simulink library "lib_ThermalManager"  (R2017a)
settings: Solver=VariableStepAuto  StartTime=0.0  StopTime=10.0  RelTol=1e-3
undefined symbols (not defined in the file): c
libraries: simulink x12
settings Model: Creator=Di Russo  LastModifiedBy=Di Russo

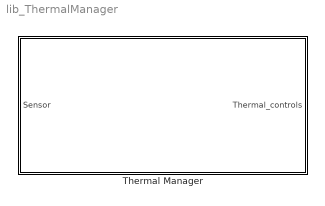
== system lib_ThermalManager ==
  Thermal Manager : Subsystem

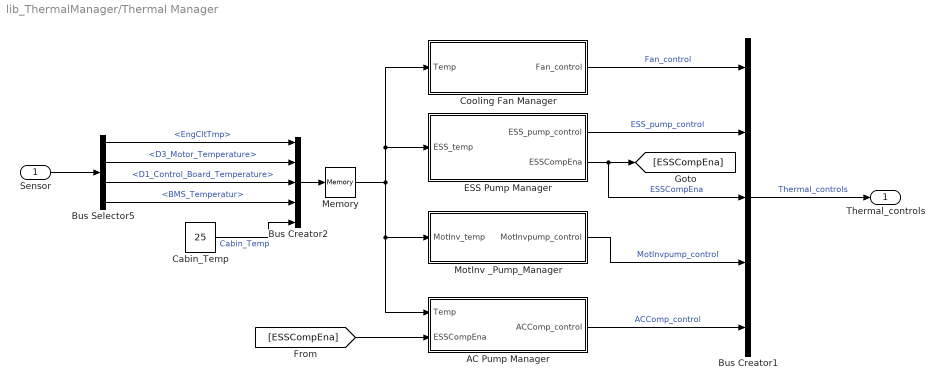
== system lib_ThermalManager/Thermal Manager ==
  Sensor : Inport
  AC Pump Manager : Subsystem
  Bus Creator1 : BusCreator  Inputs=5
  Bus Creator2 : BusCreator  Inputs=5
  Bus Selector5 : BusSelector  OutputSignals=from_CAN.fromEBCAN.from_ECM.EngCltTmp,from_CAN.fromHV_CAN.from_MCU.D3_Motor_Temperature,from_CAN.fromHV_CAN.from_MCU.D1_Control_Board_Temperature,from_CAN.fromHV_CAN.from_BMSHybrid.BMS_Temperatur
  Cabin_Temp : Constant  Value=25
  Cooling Fan Manager : Subsystem
  ESS Pump Manager : Subsystem
  Memory : Memory  X0=25
  MotInv _Pump_Manager : Subsystem
  Thermal_controls : Outport
  wires:
  Bus Creator1/1 -> Thermal_controls/1  "Thermal_controls"
  ESS Pump Manager/1(ESS_pump_control) -> Bus Creator1/2  "ESS_pump_control"
  Cooling Fan Manager/1(Fan_control) -> Bus Creator1/1  "Fan_control"
  Bus Creator2/1 -> Memory/1
  AC Pump Manager/1(ACComp_control) -> Bus Creator1/5  "ACComp_control"
  MotInv _Pump_Manager/1(MotInvpump_control) -> Bus Creator1/4  "MotInvpump_control"
  Bus Selector5/1 -> Bus Creator2/1  "<EngCltTmp>"
  Bus Selector5/2 -> Bus Creator2/2  "<D3_Motor_Temperature>"
  Bus Selector5/3 -> Bus Creator2/3  "<D1_Control_Board_Temperature>"
  Bus Selector5/4 -> Bus Creator2/4  "<BMS_Temperatur>"
  Sensor/1 -> Bus Selector5/1
  Cabin_Temp/1 -> Bus Creator2/5  "Cabin_Temp"
  ESS Pump Manager/2(ESSCompEna) -> Bus Creator1/3, [ESSCompEna]  "ESSCompEna"
  [ESSCompEna] -> AC Pump Manager/2(ESSCompEna)
  Memory/1 -> AC Pump Manager/1(Temp), MotInv _Pump_Manager/1(MotInv_temp), Cooling Fan Manager/1(Temp), ESS Pump Manager/1(ESS_temp)

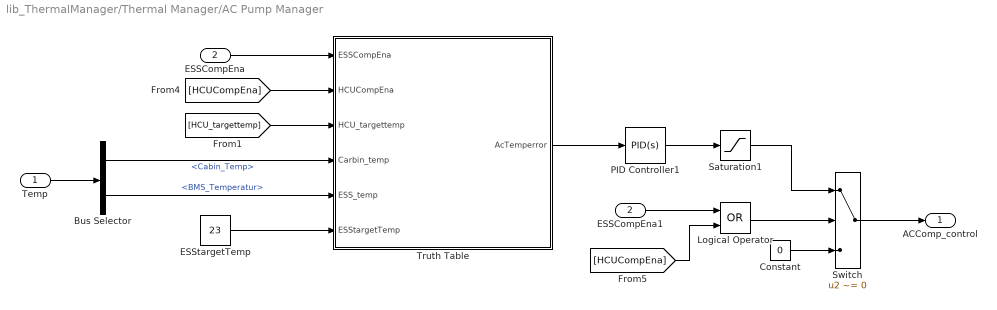
== system lib_ThermalManager/Thermal Manager/AC Pump Manager ==
  Temp : Inport
  ESSCompEna : Inport  Port=2
  Bus Selector : BusSelector  OutputSignals=Cabin_Temp,BMS_Temperatur
  Constant : Constant  Value=0
  ESSCompEna1 : InportShadow  Port=2
  ESStargetTemp : Constant  Value=23
  Logical Operator : Logic  Operator=OR  AllPortsSameDT=off  OutDataTypeStr=boolean
  PID Controller1 : simulink/Continuous/PID Controller  Controller=PID  TimeDomain=Continuous-time  SampleTime=-1  IntegratorMethod=Forward Euler  FilterMethod=Forward Euler  Form=Parallel  UseFilter=on  ControllerParametersSource=internal  P=1  I=0.01  D=0  N=100  InitialConditionSource=internal  InitialConditionForIntegrator=0  InitialConditionForFilter=0  ExternalReset=none  LimitOutput=off  UpperSaturationLimit=inf  LowerSaturationLimit=-inf  LinearizeAsGain=on  AntiWindupMode=none  Kb=1  TrackingMode=off  Kt=1  PParamMin=[]  PParamMax=[]  IParamMin=[]  IParamMax=[]  DParamMin=[]  DParamMax=[]  NParamMin=[]  NParamMax=[]  KbParamMin=[]  KbParamMax=[]  KtParamMin=[]  KtParamMax=[]  POutMin=[]  POutMax=[]  IOutMin=[]  IOutMax=[]  DOutMin=[]  DOutMax=[]  NOutMin=[]  NOutMax=[]  KbOutMin=[]  KbOutMax=[]  KtOutMin=[]  KtOutMax=[]  IntegratorOutMin=[]  IntegratorOutMax=[]  FilterOutMin=[]  FilterOutMax=[]  SumOutMin=[]  SumOutMax=[]  SumI1OutMin=[]  SumI1OutMax=[]  SumI2OutMin=[]  SumI2OutMax=[]  SumI3OutMin=[]  SumI3OutMax=[]  SumDOutMin=[]  SumDOutMax=[]  SaturationOutMin=[]  SaturationOutMax=[]  IntegratorContinuousStateAttributes=''  IntegratorStateMustResolveToSignalObject=off  IntegratorRTWStateStorageClass=Auto  FilterContinuousStateAttributes=''  FilterStateMustResolveToSignalObject=off  FilterRTWStateStorageClass=Auto  DifferentiatorICPrevScaledInput=0  DifferentiatorOutMin=[]  DifferentiatorOutMax=[]  InitialConditionSetting=State (most efficient)
  Saturation1 : Saturate  UpperLimit=1  LowerLimit=0.094
  Switch : Switch  Criteria=u2 ~= 0
  Truth Table : Truth Table  TreatAsAtomicUnit=on
  ACComp_control : Outport
  wires:
  Temp/1 -> Bus Selector/1
  PID Controller1/1 -> Saturation1/1
  Bus Selector/1 -> Truth Table/4(Carbin_temp)  "<Cabin_Temp>"
  Bus Selector/2 -> Truth Table/5(ESS_temp)  "<BMS_Temperatur>"
  ESStargetTemp/1 -> Truth Table/6(ESStargetTemp)
  Truth Table/1(AcTemperror) -> PID Controller1/1
  ESSCompEna/1 -> Truth Table/1(ESSCompEna)
  Logical Operator/1 -> Switch/2
  Constant/1 -> Switch/3
  Saturation1/1 -> Switch/1
  Switch/1 -> ACComp_control/1
  [HCU_targettemp] -> Truth Table/3(HCU_targettemp)
  [HCUCompEna] -> Truth Table/2(HCUCompEna)
  [HCUCompEna] -> Logical Operator/2
  ESSCompEna1/1 -> Logical Operator/1

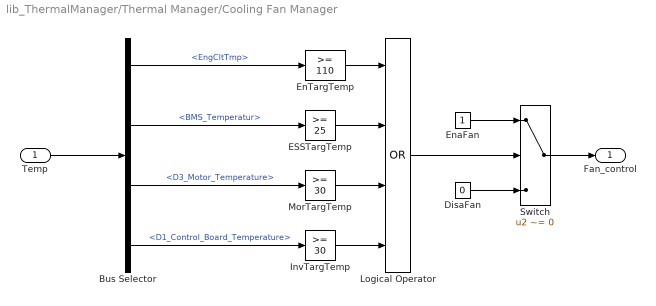
== system lib_ThermalManager/Thermal Manager/Cooling Fan Manager ==
  Temp : Inport
  Bus Selector : BusSelector  OutputSignals=EngCltTmp,BMS_Temperatur,D3_Motor_Temperature,D1_Control_Board_Temperature
  DisaFan : Constant  Value=0
  ESSTargTemp : simulink/Logic and Bit Operations/Compare To Constant  relop=>=  const=25  OutDataTypeStr=boolean
  EnTargTemp : simulink/Logic and Bit Operations/Compare To Constant  relop=>=  const=110  OutDataTypeStr=boolean
  EnaFan : Constant
  InvTargTemp : simulink/Logic and Bit Operations/Compare To Constant  relop=>=  const=30  OutDataTypeStr=boolean
  Logical Operator : Logic  Operator=OR  Inputs=4  AllPortsSameDT=off  OutDataTypeStr=boolean
  MorTargTemp : simulink/Logic and Bit Operations/Compare To Constant  relop=>=  const=30  OutDataTypeStr=boolean
  Switch : Switch  Criteria=u2 ~= 0
  Fan_control : Outport
  wires:
  Temp/1 -> Bus Selector/1
  Switch/1 -> Fan_control/1
  DisaFan/1 -> Switch/3
  Logical Operator/1 -> Switch/2
  EnaFan/1 -> Switch/1
  Bus Selector/1 -> EnTargTemp/1  "<EngCltTmp>"
  Bus Selector/2 -> ESSTargTemp/1  "<BMS_Temperatur>"
  Bus Selector/3 -> MorTargTemp/1  "<D3_Motor_Temperature>"
  Bus Selector/4 -> InvTargTemp/1  "<D1_Control_Board_Temperature>"
  EnTargTemp/1 -> Logical Operator/1
  ESSTargTemp/1 -> Logical Operator/2
  MorTargTemp/1 -> Logical Operator/3
  InvTargTemp/1 -> Logical Operator/4

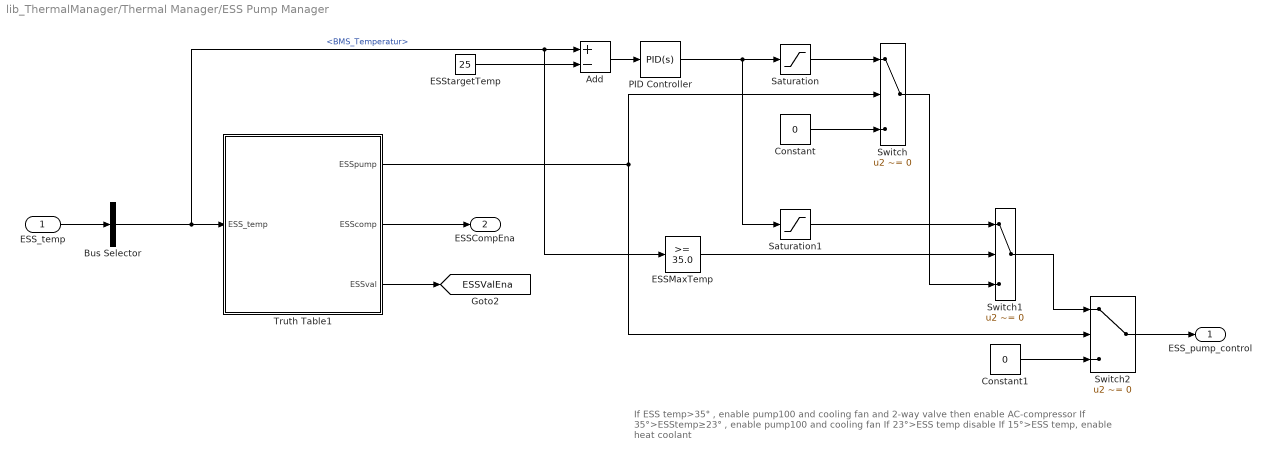
== system lib_ThermalManager/Thermal Manager/ESS Pump Manager ==
  note: If ESS temp>35°，enable pump100 and cooling fan and 2-way valve then enable AC-compressor
      |
      | If 35°>ESStemp≥23°，enable pump100 and cooling fan
      |
      | If 23°>ESS temp disable
      |
      | If 15°>ESS temp, enable heat coolant
  ESS_temp : Inport
  Add : Sum  Inputs=+-
  Bus Selector : BusSelector  OutputSignals=BMS_Temperatur
  Constant : Constant  Value=0
  Constant1 : Constant  Value=0
  ESSMaxTemp : simulink/Logic and Bit Operations/Compare To Constant  relop=>=  const=35.0  OutDataTypeStr=boolean
  ESStargetTemp : Constant  Value=25
  PID Controller : simulink/Continuous/PID Controller  Controller=PID  TimeDomain=Continuous-time  SampleTime=-1  IntegratorMethod=Forward Euler  FilterMethod=Forward Euler  Form=Parallel  UseFilter=on  ControllerParametersSource=internal  P=1  I=0.01  D=0  N=100  InitialConditionSource=internal  InitialConditionForIntegrator=0  InitialConditionForFilter=0  ExternalReset=none  LimitOutput=off  UpperSaturationLimit=inf  LowerSaturationLimit=-inf  LinearizeAsGain=on  AntiWindupMode=none  Kb=1  TrackingMode=off  Kt=1  PParamMin=[]  PParamMax=[]  IParamMin=[]  IParamMax=[]  DParamMin=[]  DParamMax=[]  NParamMin=[]  NParamMax=[]  KbParamMin=[]  KbParamMax=[]  KtParamMin=[]  KtParamMax=[]  POutMin=[]  POutMax=[]  IOutMin=[]  IOutMax=[]  DOutMin=[]  DOutMax=[]  NOutMin=[]  NOutMax=[]  KbOutMin=[]  KbOutMax=[]  KtOutMin=[]  KtOutMax=[]  IntegratorOutMin=[]  IntegratorOutMax=[]  FilterOutMin=[]  FilterOutMax=[]  SumOutMin=[]  SumOutMax=[]  SumI1OutMin=[]  SumI1OutMax=[]  SumI2OutMin=[]  SumI2OutMax=[]  SumI3OutMin=[]  SumI3OutMax=[]  SumDOutMin=[]  SumDOutMax=[]  SaturationOutMin=[]  SaturationOutMax=[]  IntegratorContinuousStateAttributes=''  IntegratorStateMustResolveToSignalObject=off  IntegratorRTWStateStorageClass=Auto  FilterContinuousStateAttributes=''  FilterStateMustResolveToSignalObject=off  FilterRTWStateStorageClass=Auto  DifferentiatorICPrevScaledInput=0  DifferentiatorOutMin=[]  DifferentiatorOutMax=[]  InitialConditionSetting=State (most efficient)
  Saturation : Saturate  UpperLimit=0.85  LowerLimit=0.13
  Saturation1 : Saturate  UpperLimit=0.97  LowerLimit=0.86
  Switch : Switch  Criteria=u2 ~= 0
  Switch1 : Switch  Criteria=u2 ~= 0  Threshold=1
  Switch2 : Switch  Criteria=u2 ~= 0  Threshold=c
  Truth Table1 : Truth Table  TreatAsAtomicUnit=on
  ESS_pump_control : Outport
  ESSCompEna : Outport  Port=2
  tag scope: ESSValEna=global
  wires:
  Truth Table1/1(ESSpump) -> Switch2/2, Switch/2
  ESS_temp/1 -> Bus Selector/1
  Bus Selector/1 -> ESSMaxTemp/1, Add/1, Truth Table1/1(ESS_temp)  "<BMS_Temperatur>"
  Constant/1 -> Switch/3
  PID Controller/1 -> Saturation1/1, Saturation/1
  Add/1 -> PID Controller/1
  Saturation/1 -> Switch/1
  ESSMaxTemp/1 -> Switch1/2
  ESStargetTemp/1 -> Add/2
  Truth Table1/2(ESScomp) -> ESSCompEna/1
  Truth Table1/3(ESSval) -> [ESSValEna]
  Constant1/1 -> Switch2/3
  Switch2/1 -> ESS_pump_control/1
  Switch1/1 -> Switch2/1
  Switch/1 -> Switch1/3
  Saturation1/1 -> Switch1/1

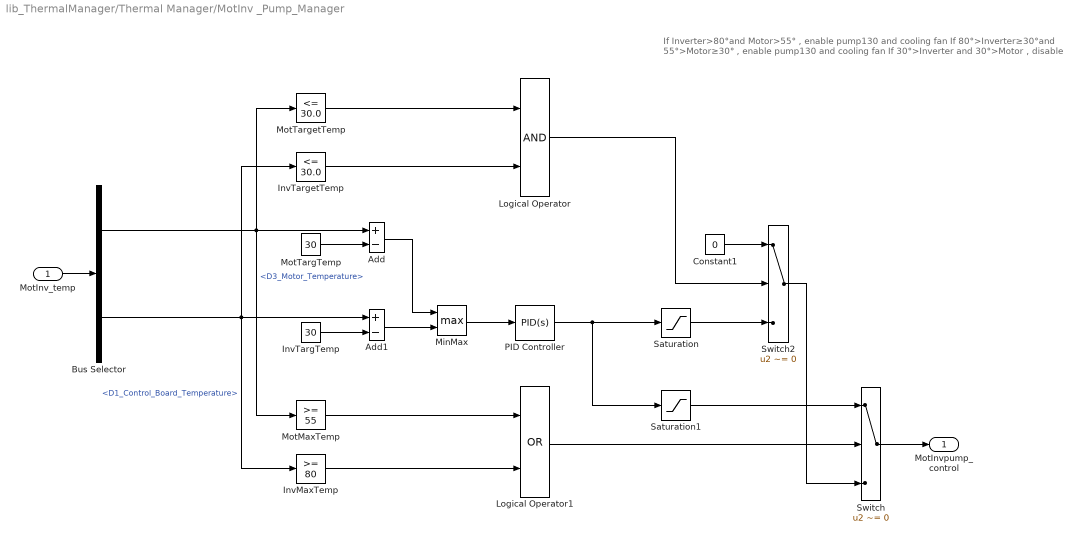
== system lib_ThermalManager/Thermal Manager/MotInv _Pump_Manager ==
  note: If Inverter>80°and Motor>55°，enable pump130 and cooling fan
      |
      | If 80°>Inverter≥30°and 55°>Motor≥30°，enable pump130 and cooling fan
      |
      | If 30°>Inverter and 30°>Motor，disable
  MotInv_temp : Inport
  Add : Sum  Inputs=+-
  Add1 : Sum  Inputs=+-
  Bus Selector : BusSelector  OutputSignals=D3_Motor_Temperature,D1_Control_Board_Temperature
  Constant1 : Constant  Value=0
  InvMaxTemp : simulink/Logic and Bit Operations/Compare To Constant  relop=>=  const=80  OutDataTypeStr=boolean
  InvTargTemp : Constant  Value=30
  InvTargetTemp : simulink/Logic and Bit Operations/Compare To Constant  relop=<=  const=30.0  OutDataTypeStr=boolean
  Logical Operator : Logic  AllPortsSameDT=off  OutDataTypeStr=boolean
  Logical Operator1 : Logic  Operator=OR  AllPortsSameDT=off  OutDataTypeStr=boolean
  MinMax : MinMax  Function=max  Inputs=2
  MotMaxTemp : simulink/Logic and Bit Operations/Compare To Constant  relop=>=  const=55  OutDataTypeStr=boolean
  MotTargTemp : Constant  Value=30
  MotTargetTemp : simulink/Logic and Bit Operations/Compare To Constant  relop=<=  const=30.0  OutDataTypeStr=boolean
  PID Controller : simulink/Continuous/PID Controller  Controller=PID  TimeDomain=Continuous-time  SampleTime=-1  IntegratorMethod=Forward Euler  FilterMethod=Forward Euler  Form=Parallel  UseFilter=on  ControllerParametersSource=internal  P=0.05  I=0.001  D=5  N=100  InitialConditionSource=internal  InitialConditionForIntegrator=0  InitialConditionForFilter=0  ExternalReset=none  LimitOutput=off  UpperSaturationLimit=inf  LowerSaturationLimit=-inf  LinearizeAsGain=on  AntiWindupMode=none  Kb=1  TrackingMode=off  Kt=1  PParamMin=[]  PParamMax=[]  IParamMin=[]  IParamMax=[]  DParamMin=[]  DParamMax=[]  NParamMin=[]  NParamMax=[]  KbParamMin=[]  KbParamMax=[]  KtParamMin=[]  KtParamMax=[]  POutMin=[]  POutMax=[]  IOutMin=[]  IOutMax=[]  DOutMin=[]  DOutMax=[]  NOutMin=[]  NOutMax=[]  KbOutMin=[]  KbOutMax=[]  KtOutMin=[]  KtOutMax=[]  IntegratorOutMin=[]  IntegratorOutMax=[]  FilterOutMin=[]  FilterOutMax=[]  SumOutMin=[]  SumOutMax=[]  SumI1OutMin=[]  SumI1OutMax=[]  SumI2OutMin=[]  SumI2OutMax=[]  SumI3OutMin=[]  SumI3OutMax=[]  SumDOutMin=[]  SumDOutMax=[]  SaturationOutMin=[]  SaturationOutMax=[]  IntegratorContinuousStateAttributes=''  IntegratorStateMustResolveToSignalObject=off  IntegratorRTWStateStorageClass=Auto  FilterContinuousStateAttributes=''  FilterStateMustResolveToSignalObject=off  FilterRTWStateStorageClass=Auto  DifferentiatorICPrevScaledInput=0  DifferentiatorOutMin=[]  DifferentiatorOutMax=[]  InitialConditionSetting=State (most efficient)
  Saturation : Saturate  UpperLimit=0.85  LowerLimit=0.13
  Saturation1 : Saturate  UpperLimit=0.97  LowerLimit=0.86
  Switch : Switch  Criteria=u2 ~= 0  Threshold=1
  Switch2 : Switch  Criteria=u2 ~= 0  Threshold=1
  MotInvpump_control : Outport
  wires:
  MotInv_temp/1 -> Bus Selector/1
  Bus Selector/1 -> MotTargetTemp/1, Add/1, MotMaxTemp/1  "<D3_Motor_Temperature>"
  Bus Selector/2 -> InvTargetTemp/1, InvMaxTemp/1, Add1/1  "<D1_Control_Board_Temperature>"
  MotTargetTemp/1 -> Logical Operator/1
  InvTargetTemp/1 -> Logical Operator/2
  Add/1 -> MinMax/1
  Add1/1 -> MinMax/2
  MinMax/1 -> PID Controller/1
  PID Controller/1 -> Saturation1/1, Saturation/1
  Logical Operator/1 -> Switch2/2
  MotMaxTemp/1 -> Logical Operator1/1
  InvMaxTemp/1 -> Logical Operator1/2
  Logical Operator1/1 -> Switch/2
  Switch/1 -> MotInvpump_control/1
  MotTargTemp/1 -> Add/2
  InvTargTemp/1 -> Add1/2
  Switch2/1 -> Switch/3
  Saturation1/1 -> Switch/1
  Saturation/1 -> Switch2/3
  Constant1/1 -> Switch2/1

== matlab function lib_ThermalManager/Thermal Manager/AC Pump Manager/Truth Table ==
  data: ESSCompEna input; AcTemperror output; HCUCompEna input double; HCU_targettemp input double; Carbin_temp input double; ESS_temp input double; ESStargetTemp input double
function AcTemperror = fcn(ESSCompEna, HCUCompEna, HCU_targettemp, Carbin_temp, ESS_temp, ESStargetTemp)

aVarTruthTableCondition_1 = false;
aVarTruthTableCondition_2 = false;
aVarTruthTableCondition_3 = false;
aVarTruthTableCondition_4 = false;


% Disable comp

aVarTruthTableCondition_1 = logical(ESSCompEna==0 && HCUCompEna==0);

% ESS enable HCU disable

aVarTruthTableCondition_2 = logical(ESSCompEna==1 && HCUCompEna==0);

% ESS disable HCU enable

aVarTruthTableCondition_3 = logical(ESSCompEna==0 && HCUCompEna==1);

% ESS enable HCU enable

aVarTruthTableCondition_4 = logical(ESSCompEna==1 && HCUCompEna==1);

if (aVarTruthTableCondition_1 && aVarTruthTableCondition_2 && ~aVarTruthTableCondition_3 && ~aVarTruthTableCondition_4)
    aFcnTruthTableAction_1();
elseif (~aVarTruthTableCondition_1 && aVarTruthTableCondition_2 && ~aVarTruthTableCondition_3 && ~aVarTruthTableCondition_4)
    aFcnTruthTableAction_2();
elseif (~aVarTruthTableCondition_1 && ~aVarTruthTableCondition_2 && aVarTruthTableCondition_3 && ~aVarTruthTableCondition_4)
    aFcnTruthTableAction_3();
elseif (~aVarTruthTableCondition_1 && ~aVarTruthTableCondition_2 && ~aVarTruthTableCondition_3 && aVarTruthTableCondition_4)
    aFcnTruthTableAction_4();
else % Default
    aFcnTruthTableAction_5();
end

function aFcnTruthTableAction_1()

% AC Compressor output condition1

AcTemperror = 0;

function aFcnTruthTableAction_2()

% AC Compressor output condition2

AcTemperror = ESS_temp - ESStargetTemp;

function aFcnTruthTableAction_3()

% AC Compressor output condition3

AcTemperror = Carbin_temp - HCU_targettemp;

function aFcnTruthTableAction_4()

% AC Compressor output condition4

AcTemperror = ESS_temp - ESStargetTemp + Carbin_temp - HCU_targettemp;

function aFcnTruthTableAction_5()

% Defaut

AcTemperror = 0;

== matlab function lib_ThermalManager/Thermal Manager/ESS Pump Manager/Truth Table1 ==
  data: ESSpump output double; ESS_temp input double; ESScomp output double; ESSval output double
function [ESSpump, ESScomp, ESSval] = fcn(ESS_temp)

aVarTruthTableCondition_1 = false;
aVarTruthTableCondition_2 = false;
aVarTruthTableCondition_3 = false;
aVarTruthTableCondition_4 = false;


% enable pump and AC compr

aVarTruthTableCondition_1 = logical(ESS_temp >= 35);

% enable pump and disable AC compr

aVarTruthTableCondition_2 = logical(ESS_temp < 35 && ESS_temp >= 23);

% disable pump and AC compr

aVarTruthTableCondition_3 = logical(ESS_temp < 23 && ESS_temp >= 15);

% heating

aVarTruthTableCondition_4 = logical(ESS_temp < 15);

if (aVarTruthTableCondition_1 && ~aVarTruthTableCondition_2 && ~aVarTruthTableCondition_3 && ~aVarTruthTableCondition_4)
    aFcnTruthTableAction_1();
elseif (~aVarTruthTableCondition_1 && aVarTruthTableCondition_2 && ~aVarTruthTableCondition_3 && ~aVarTruthTableCondition_4)
    aFcnTruthTableAction_2();
elseif (~aVarTruthTableCondition_1 && ~aVarTruthTableCondition_2 && aVarTruthTableCondition_3 && ~aVarTruthTableCondition_4)
    aFcnTruthTableAction_3();
elseif (~aVarTruthTableCondition_1 && ~aVarTruthTableCondition_2 && ~aVarTruthTableCondition_3 && aVarTruthTableCondition_4)
    aFcnTruthTableAction_4();
else % Default
    aFcnTruthTableAction_5();
end

function aFcnTruthTableAction_1()

% ESS_temp request case1

ESSpump=1; ESScomp=1; ESSval=1;

function aFcnTruthTableAction_2()

% ESS_temp request case2

ESSpump=1; ESScomp=0; ESSval=0;

function aFcnTruthTableAction_3()

% ESS_temp request case3

ESSpump=0; ESScomp=0; ESSval=0;

function aFcnTruthTableAction_4()

% ESS_temp request case4

ESSpump=0; ESScomp=0; ESSval=0;

function aFcnTruthTableAction_5()

% Default

ESSpump=0; ESScomp=0; ESSval=0;
